simulink model "s_to_N"  (R2025b)
settings: Solver=FixedStepAuto  StartTime=0.0  StopTime=10.0  RelTol=1e-3
settings Model: Creator=Huawei  LastModifiedBy=lolve
settings OptimizationCC: BlockReduction=off  UseDivisionForNetSlopeComputation=on  OptimizeBlockIOStorage=off

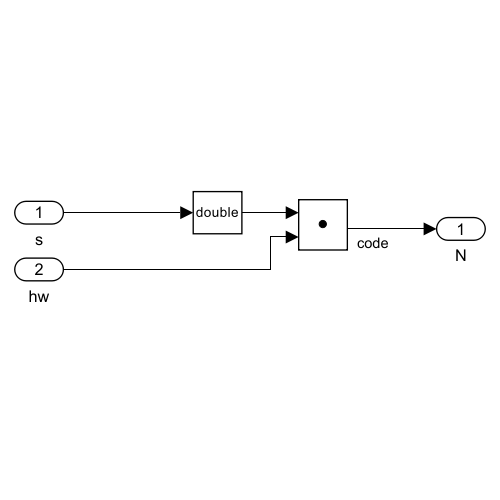
[thumbnail: Simulink's stored preview of the top-level diagram]
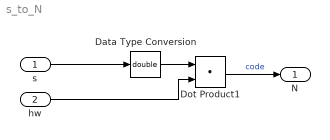
== system s_to_N ==
  s : Inport  OutDataTypeStr=uint16  PortDimensions=5000
  hw : Inport  Port=2  PortDimensions=5000
  Data Type Conversion : DataTypeConversion  OutDataTypeStr=double  SaturateOnIntegerOverflow=off  RndMeth=Floor
  Dot Product1 : DotProduct  OutDataTypeStr=Inherit: Inherit via internal rule
  N : Outport
  wires:
  s/1 -> Data Type Conversion/1
  Data Type Conversion/1 -> Dot Product1/1
  hw/1 -> Dot Product1/2
  Dot Product1/1 -> N/1  "code"
